simulink model "modelSimple"  (R2023b)
settings: Solver=FixedStepAuto  StartTime=0.0  StopTime=inf  FixedStep=0.01  RelTol=1e-3
model workspace (MAT data in the model file):
  freq = 0.87
settings Model: Creator=marko  LastModifiedBy=marko
settings DebuggingCC: UnconnectedInputMsg=warning  UnconnectedOutputMsg=warning  UnconnectedLineMsg=warning
settings ModelReferenceCC: EnableRefExpFcnMdlSchedulingChecks=on
settings RTWCC: DLArmComputeVersion=19.05
settings ConfigComp: CovBoundaryAbsTol=1.0e-5

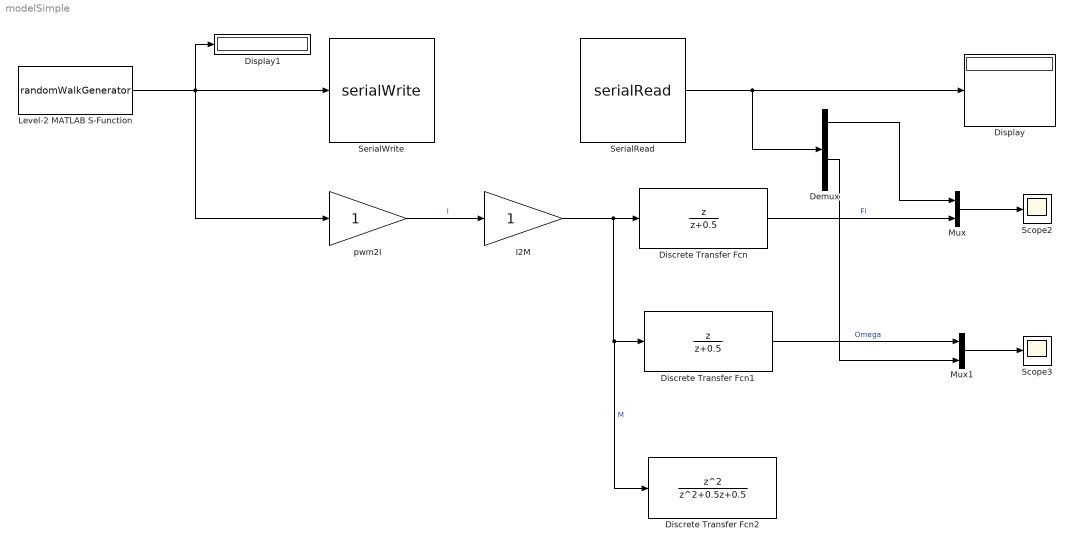
== system modelSimple ==
  Demux : Demux
  Discrete Transfer Fcn : DiscreteTransferFcn  Numerator=[1 0]
  Discrete Transfer Fcn1 : DiscreteTransferFcn  Numerator=[1 0]
  Discrete Transfer Fcn2 : DiscreteTransferFcn  Numerator=[1 0 0]  Denominator=[1 0.5 0.5]
  Display : Display
  Display1 : Display
  I2M : Gain
  Level-2 MATLAB S-Function : M-S-Function  FunctionName=randomWalkGenerator
  Mux : Mux  Inputs=2
  Mux1 : Mux  Inputs=2
  Scope2 : Scope
  Scope3 : Scope
  SerialRead : M-S-Function  FunctionName=serialRead  Parameters='COM4'
  SerialWrite : M-S-Function  FunctionName=serialWrite  Parameters='COM4'
  pwm2I : Gain
  wires:
  SerialRead/1 -> Demux/1, Display/1
  Level-2 MATLAB S-Function/1 -> Display1/1, pwm2I/1, SerialWrite/1
  Discrete Transfer Fcn/1 -> Mux/2  "Fi"
  pwm2I/1 -> I2M/1  "I"
  I2M/1 -> Discrete Transfer Fcn2/1, Discrete Transfer Fcn1/1, Discrete Transfer Fcn/1  "M"
  Discrete Transfer Fcn1/1 -> Mux1/1  "Omega"
  Demux/1 -> Mux/1
  Demux/3 -> Mux1/2
  Mux/1 -> Scope2/1
  Mux1/1 -> Scope3/1
